simulink model "prelab"  (R2019b)
settings: Solver=VariableStepAuto  StartTime=0.0  StopTime=10.0  RelTol=1e-3
settings Model: Creator=tangj  LastModifiedBy=tangj

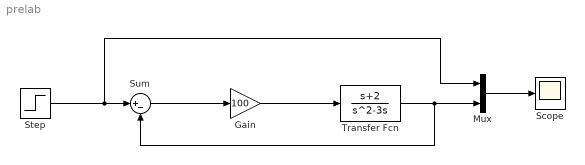
== system prelab ==
  Gain : Gain  Gain=100
  Mux : Mux  Inputs=2
  Scope : Scope
  Step : Step  SampleTime=0
  Sum : Sum  Inputs=|+-
  Transfer Fcn : TransferFcn  Numerator=[0,1,2]  Denominator=[1 -3 0]
  wires:
  Gain/1 -> Transfer Fcn/1
  Sum/1 -> Gain/1
  Step/1 -> Mux/1, Sum/1
  Mux/1 -> Scope/1
  Transfer Fcn/1 -> Sum/2, Mux/2
